simulink model "psbconverter"  (Simulink 6.0)
settings: Solver=ode15s  SolverMode=SingleTasking  StartTime=0.0  StopTime=.1  RelTol=1e-2  AbsTol=1e-3
InitFcn:
  | powericon('psbinitsys',bdroot);
libraries: powerlib2 x21, powerlib_extras x1
settings Model: Creator=sybille  LastModifiedBy=batserve  ExtModeTrigMode=oneshot  ExtModeArmWhenConnect=off  ExtModeAutoUpdateStatusClock=off
settings SolverCC: MaxOrder=1
settings DataIOCC: LimitDataPoints=off  SaveOutput=off  SaveTime=off  SignalLoggingName=sigsOut
settings OptimizationCC: BlockReduction=off  BooleanDataType=off
settings DebuggingCC: CheckExecutionContextPreStartOutputMsg=on  CheckExecutionContextRuntimeOutputMsg=on  SolverPrmCheckMsg=none  UnconnectedInputMsg=none  UnconnectedOutputMsg=none
settings HardwareCC: TargetUnknown=on
settings RTWCC: TemplateMakefile=grt_unix.tmf

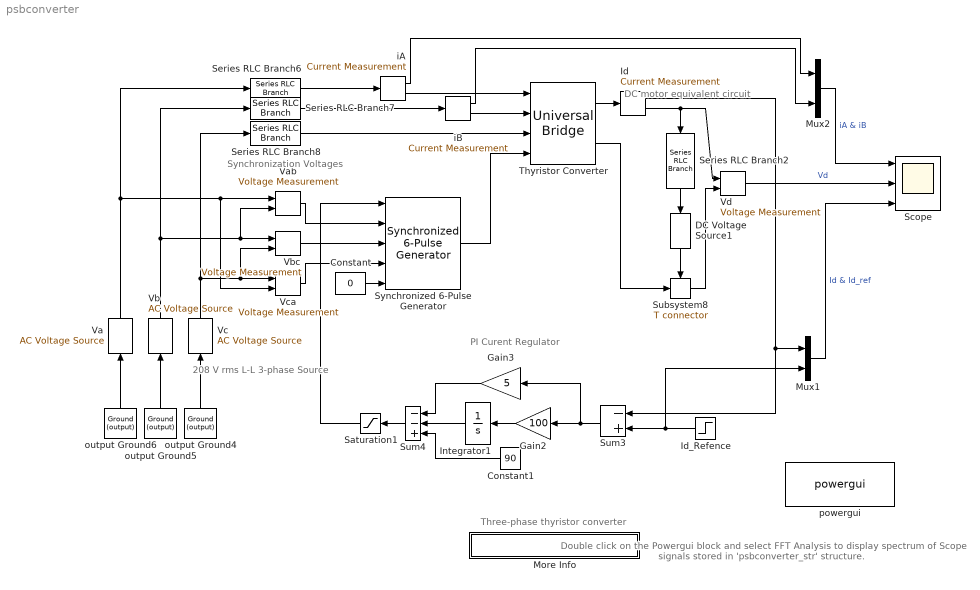
== system psbconverter ==
  note: Synchronization Voltages
  note: DC motor equivalent circuit
  note: PI Curent Regulator
  note: Three-phase thyristor converter
  note: 208 V rms L-L
      | 3-phase Source
  note: Double click on the Powergui block
      | and select FFT Analysis to display
      | spectrum of Scope  signals stored in
      | 'psbconverter_str' structure.
  Constant : Constant  Value=0
  Constant1 : Constant  Orientation=left  Value=90
  DC Voltage Source1 : powerlib2/Electrical Sources/DC Voltage Source  Tag=PoWeRsYsTeMbLoCk  Orientation=down  V=-120  mesure=None  PSBOutputType=1
  Gain2 : Gain  Orientation=left  Gain=100  SaturateOnIntegerOverflow=on
  Gain3 : Gain  Orientation=left  Gain=5  SaturateOnIntegerOverflow=on
  Id : powerlib2/Measurements/Current Measurement  Tag=PoWeRsYsTeMmEaSuReMeNt  PhasorSimulation=off  OutputType=Complex  PSBOutputType=01  PSBequivalent=0
  Id_Refence : Step  Orientation=left  Time=0.04  Before=10  After=25  SampleTime=0
  Integrator1 : Integrator  Orientation=left  InitialCondition=20  LimitOutput=on  UpperSaturationLimit=160  LowerSaturationLimit=20
  More Info : Subsystem
      mask Display: disp('? : Double click here for more info ')
  Mux1 : Mux  Inputs=2
  Mux2 : Mux  Inputs=2
  Saturation1 : Saturate  Orientation=left  UpperLimit=160  LowerLimit=20
  Scope : Scope  NumInputPorts=3
      settings: TimeRange=0.1  YMin=-50~-200~-3.202157228752688e-017  YMax=50~400~40  SaveName=psbconverter_str  SampleInput=on  SampleTime=1/60/512
  Series RLC Branch2 : powerlib2/Elements/Series RLC Branch  Tag=PoWeRsYsTeMbLoCk  Orientation=down  a=1  b=20e-3  c=inf  mesure=None  PSBOutputType=1
  Series RLC Branch6 : powerlib2/Elements/Series RLC Branch  Tag=PoWeRsYsTeMbLoCk  a=0.01  b=1e-3  c=inf  mesure=None  PSBOutputType=1
  Series RLC Branch7 : powerlib2/Elements/Series RLC Branch  Tag=PoWeRsYsTeMbLoCk  a=0.01  b=1e-3  c=inf  mesure=None  PSBOutputType=1
  Series RLC Branch8 : powerlib2/Elements/Series RLC Branch  Tag=PoWeRsYsTeMbLoCk  a=0.01  b=1e-3  c=inf  mesure=None  PSBOutputType=1
  Subsystem8 : powerlib2/Connectors/T connector  Tag=PoWeRsYsTeMbLoCk  PSBOutputType=1
  Sum3 : Sum  Orientation=left  Inputs=-+  SaturateOnIntegerOverflow=on  InputSameDT=on
  Sum4 : Sum  Orientation=left  Inputs=--+  SaturateOnIntegerOverflow=on  InputSameDT=on
  Synchronized 6-Pulse Generator : powerlib_extras/Control  Blocks/Synchronized 6-Pulse Generator  freq=60  pwidth=10  Double_Pulse=on
  Thyristor Converter : powerlib2/Power Electronics/Universal Bridge  Tag=PoWeRsYsTeMbLoCk  arms=3  confi=ABC as input terminals  injcc=500  cf=.1e-6  device=Thyristors  Ron=1e-3  Lon=0  VFs="[  0.8  0.8  ]"  Vf=.8  gtoparameters=[ 10e-6 , 20e-6 ]  igbtparameters=[ 1e-6 , 2e-6 ]  mesure=None  PSBOutputType=111
  Va : powerlib2/Electrical Sources/AC Voltage Source  Tag=PoWeRsYsTeMbLoCk  Orientation=up  A=208*sqrt(2/3)  P=0  F=60  stime=0  mesure=None  PSBOutputType=1
  Vab : powerlib2/Measurements/Voltage Measurement  Tag=PoWeRsYsTeMmEaSuReMeNt  PhasorSimulation=off  OutputType=Complex  PSBOutputType=0  PSBequivalent=0
  Vb : powerlib2/Electrical Sources/AC Voltage Source  Tag=PoWeRsYsTeMbLoCk  Orientation=up  A=208*sqrt(2/3)  P=-120  F=60  stime=0  mesure=None  PSBOutputType=1
  Vbc : powerlib2/Measurements/Voltage Measurement  Tag=PoWeRsYsTeMmEaSuReMeNt  PhasorSimulation=off  OutputType=Complex  PSBOutputType=0  PSBequivalent=0
  Vc : powerlib2/Electrical Sources/AC Voltage Source  Tag=PoWeRsYsTeMbLoCk  Orientation=up  A=208*sqrt(2/3)  P=120  F=60  stime=0  mesure=None  PSBOutputType=1
  Vca : powerlib2/Measurements/Voltage Measurement  Tag=PoWeRsYsTeMmEaSuReMeNt  PhasorSimulation=off  OutputType=Complex  PSBOutputType=0  PSBequivalent=0
  Vd : powerlib2/Measurements/Voltage Measurement  Tag=PoWeRsYsTeMmEaSuReMeNt  PhasorSimulation=off  OutputType=Complex  PSBOutputType=0  PSBequivalent=0
  iA : powerlib2/Measurements/Current Measurement  Tag=PoWeRsYsTeMmEaSuReMeNt  PhasorSimulation=off  OutputType=Complex  PSBOutputType=01  PSBequivalent=0
  iB : powerlib2/Measurements/Current Measurement  Tag=PoWeRsYsTeMmEaSuReMeNt  PhasorSimulation=off  OutputType=Complex  PSBOutputType=01  PSBequivalent=0
  output Ground4 : powerlib2/Connectors/Ground (output)  Tag=PoWeRsYsTeMbLoCk  Orientation=up  PSBOutputType=1
  output Ground5 : powerlib2/Connectors/Ground (output)  Tag=PoWeRsYsTeMbLoCk  Orientation=up  PSBOutputType=1
  output Ground6 : powerlib2/Connectors/Ground (output)  Tag=PoWeRsYsTeMbLoCk  Orientation=up  PSBOutputType=1
  powergui : powerlib2/powergui  Frange=[0:2:500]  Ylog=off  Xlog=on  save=off  variable=ZData  structure=psbconverter_str  ZoomFFT=on  StartTime=0.1-2/60  cycles=2  DisplayStyle=off  fundamental=60  FreqAxis=on  MaxFrequency=2000  frequencyindice=1  frequencyindicesteady=1  RmsSteady=1  display=off  Ts=0  methode=off  frequency=60  echomessages=off
  wires:
  Thyristor Converter/1 -> Id/1
  output Ground6/1 -> Va/1
  output Ground5/1 -> Vb/1
  output Ground4/1 -> Vc/1
  Thyristor Converter/2 -> Subsystem8/1
  Subsystem8/1 -> Vd/2
  Id/2 -> Series RLC Branch2/1, Vd/1
  Series RLC Branch2/1 -> DC Voltage Source1/1
  DC Voltage Source1/1 -> Subsystem8/Enable
  Gain3/1 -> Sum4/1
  Constant1/1 -> Sum4/3
  Gain2/1 -> Integrator1/1
  Sum3/1 -> Gain3/1, Gain2/1
  Sum4/1 -> Saturation1/1
  Id/1 -> Mux1/1, Sum3/1
  Integrator1/1 -> Sum4/2
  Vb/1 -> Vbc/1, Vab/2, Series RLC Branch7/1
  Vc/1 -> Vca/1, Vbc/2, Series RLC Branch8/1
  Va/1 -> Vab/1, Vca/2, Series RLC Branch6/1
  Vca/1 -> Synchronized 6-Pulse Generator/4
  Vbc/1 -> Synchronized 6-Pulse Generator/3
  Vab/1 -> Synchronized 6-Pulse Generator/2
  Series RLC Branch8/1 -> Thyristor Converter/3
  Saturation1/1 -> Synchronized 6-Pulse Generator/1
  Id_Refence/1 -> Sum3/2, Mux1/2
  Series RLC Branch6/1 -> iA/1
  iA/2 -> Thyristor Converter/1
  Series RLC Branch7/1 -> iB/1
  iB/2 -> Thyristor Converter/2
  iA/1 -> Mux2/1
  iB/1 -> Mux2/2
  Mux2/1 -> Scope/1  "iA & iB"
  Vd/1 -> Scope/2  "Vd"
  Mux1/1 -> Scope/3  "Id & Id_ref"
  Constant/1 -> Synchronized 6-Pulse Generator/5
  Synchronized 6-Pulse Generator/1 -> Thyristor Converter/4

== system psbconverter/More Info ==
  note: This demonstration illustrates use of the Universal Bridge block to simulate a three-phase six-pulse
      | converter and harmonic analysis using the Powergui/FFT tool.
  note: Circuit Description
  note: A  DC motor  represented by a simplified RL-E model is fed from  an inductive three-phase source through a six-pulse
      | thyristor bridge. A pulse generator synchronized on the source voltages provides the trigger pulses for the six thyristors.
      |
      | The converter output current is controlled by a PI current regulator built with Simulink blocks.
      | A step signal is applied to the reference input to test the dynamic response of the current regulator.
      |
      | In order to allow further signal processing, signals displayed on the Scope block are sampled at 1/60/512 s (512 samples/ cycle) and stored
      | in a variable named 'psbconveter_str'  ('structure with time'  format) .
  note: H. Le-Huy (Universite Laval, Quebec)
  note: Demonstration
  note: Start simulation and observe current and voltage waveforms on the Scope block.
      |
      | When  simulation is completed, open the Powergui and select  'FFT Analysis' to display the 0 - 2000 Hz frequency spectrum of signals saved
      | in the 'psbconverter_str' structure. The FFT will be performed on  a 2-cycle window starting at t = 0.1 - 2/60 (last 2 cycles of recording).
      | Input labeled 'Ia & Ib' and signal number 1 (Ia) should be already selected. Click on Display and observe the frequency spectrum of last two cycles of Ia.
      | Harmonic currents (6n+/-1) are displayed in % of the fundamental component .
      |
      | The value of the fundamental current (magnitude = 27.48 A peak) and the Total Harmonic Distortion (THD) are also displayed.
      | Harrmonics in the 0 - 2000 Hz range contribute to 29% in THD. If you specify a 0-4000 Hz frequence range you will notice that
      | contribution of harmonics above 2000 Hz is negligible in the current THD.
      |
      | Now select input labeled Vd and display its spectrum.
      | The DC voltage contains harmonics (6n) and its DC component is 145.4 V.
